simulink model "P_I_PI_Controllers"  (R2023b)
settings: Solver=VariableStepAuto  StartTime=0.0  StopTime=30  MaxStep=1e-3  RelTol=1e-3
settings Model: Creator=MOHAMED  LastModifiedBy=MOHAMED

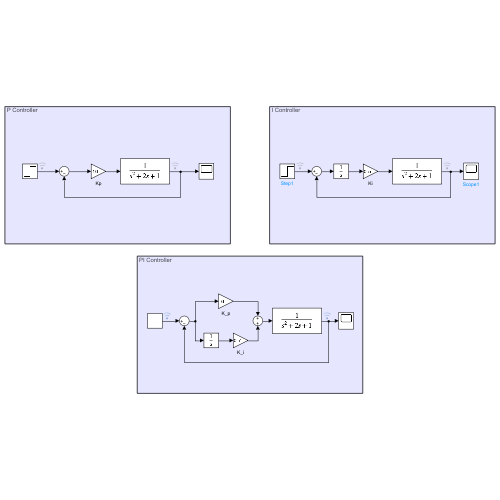
[thumbnail: Simulink's stored preview of the top-level diagram]
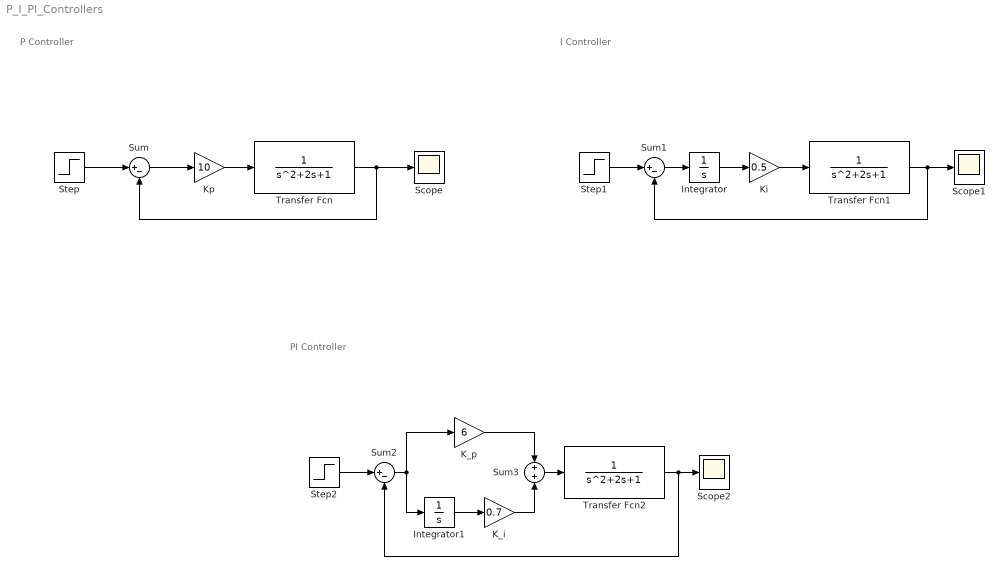
== system P_I_PI_Controllers ==
  note: P Controller
  note: I Controller
  note: PI Controller
  Integrator : Integrator
  Integrator1 : Integrator
  K_i : Gain  Gain=0.7
  K_p : Gain  Gain=6
  Ki : Gain  Gain=0.5
  Kp : Gain  Gain=10
  Scope : Scope
  Scope1 : Scope
  Scope2 : Scope
  Step : Step  SampleTime=0
  Step1 : Step  SampleTime=0
  Step2 : Step  SampleTime=0
  Sum : Sum  Inputs=|+-
  Sum1 : Sum  Inputs=|+-
  Sum2 : Sum  Inputs=|+-
  Sum3 : Sum
  Transfer Fcn : TransferFcn
  Transfer Fcn1 : TransferFcn
  Transfer Fcn2 : TransferFcn
  wires:
  Transfer Fcn/1 -> Sum/2, Scope/1
  Step/1 -> Sum/1
  Sum/1 -> Kp/1
  Kp/1 -> Transfer Fcn/1
  Ki/1 -> Transfer Fcn1/1
  Sum1/1 -> Integrator/1
  Step1/1 -> Sum1/1
  Transfer Fcn1/1 -> Sum1/2, Scope1/1
  Integrator/1 -> Ki/1
  Integrator1/1 -> K_i/1
  Transfer Fcn2/1 -> Sum2/2, Scope2/1
  Step2/1 -> Sum2/1
  Sum2/1 -> K_p/1, Integrator1/1
  Sum3/1 -> Transfer Fcn2/1
  K_i/1 -> Sum3/2
  K_p/1 -> Sum3/1
